simulink model "bh_integration_concept"  (R2017a)
settings: Solver=ode45  StartTime=0.0  StopTime=10  MaxStep=0.01  RelTol=1e-5  EnableMultiTasking=on
settings Model: Creator=bhorton  LastModifiedBy=bhorton
settings OptimizationCC: LifeSpan=inf
settings DebuggingCC: SFUnexpectedBacktrackingDiag=warning  SFNoUnconditionalDefaultTransitionDiag=warning  SFExecutionAtInitializationDiag=none
settings GRTTargetCC: TargetLangStandard=C89/C90 (ANSI)  GeneratePreprocessorConditionals=Disable all
settings ConfigComp: CovMetricSettings=dw  CovHtmlReporting=on  CovSaveCumulativeToWorkspaceVar=on  CovSaveSingleToWorkspaceVar=on  CovExternalEMLEnable=off

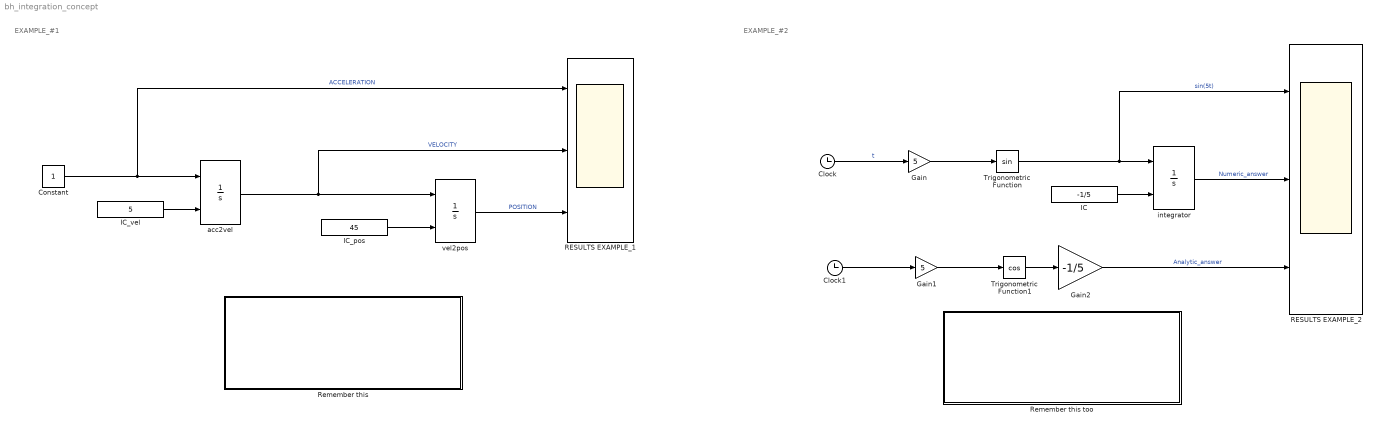
== system bh_integration_concept ==
  note: EXAMPLE_#2
  note: EXAMPLE_#1
  Clock : Clock
  Clock1 : Clock
  Constant : Constant
  Gain : Gain  Gain=5
  Gain1 : Gain  Gain=5
  Gain2 : Gain  Gain=-1/5
  IC : Constant  Value=-1/5
  IC_pos : Constant  Value=45
  IC_vel : Constant  Value=5
  RESULTS EXAMPLE_1 : Scope  NumInputPorts=3
  RESULTS EXAMPLE_2 : Scope  NumInputPorts=3
  Remember this : Subsystem
  Remember this too : Subsystem
  Trigonometric Function : Trigonometry
  Trigonometric Function1 : Trigonometry  Operator=cos
  acc2vel : Integrator  InitialConditionSource=external
  integrator : Integrator  InitialConditionSource=external
  vel2pos : Integrator  InitialConditionSource=external
  wires:
  Constant/1 -> RESULTS EXAMPLE_1/1, acc2vel/1  "ACCELERATION"
  acc2vel/1 -> RESULTS EXAMPLE_1/2, vel2pos/1  "VELOCITY"
  vel2pos/1 -> RESULTS EXAMPLE_1/3  "POSITION"
  IC_vel/1 -> acc2vel/2
  IC_pos/1 -> vel2pos/2
  IC/1 -> integrator/2
  Trigonometric Function/1 -> RESULTS EXAMPLE_2/1, integrator/1  "sin(5t)"
  integrator/1 -> RESULTS EXAMPLE_2/2  "Numeric_answer"
  Clock/1 -> Gain/1  "t"
  Gain/1 -> Trigonometric Function/1
  Clock1/1 -> Gain1/1
  Gain1/1 -> Trigonometric Function1/1
  Trigonometric Function1/1 -> Gain2/1
  Gain2/1 -> RESULTS EXAMPLE_2/3  "Analytic_answer"

== system bh_integration_concept/Remember this ==

== system bh_integration_concept/Remember this too ==
  note: We all know the following INDEFINITE integral:
  note: And we can also write this as a DEFINITE integral:
